simulink model "example"  (R2021a)
settings: Solver=VariableStepAuto  StartTime=0.0  StopTime=10.0  RelTol=1e-3
settings Model: Creator=ibirl  LastModifiedBy=zht

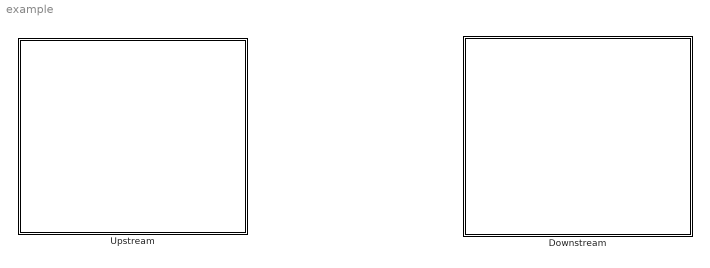
== system example ==
  Downstream : Stateflow chart  TreatAsAtomicUnit=on
  Upstream : Stateflow chart  TreatAsAtomicUnit=on

== stateflow chart example/Downstream ==
  state AFailed
  state BOperational
  state CStarved
  state DDelayed
  AFailed -> AFailed [order 3] : (1)[1-p3]{0}
  DDelayed -> AFailed [order 2] : (1)[p4]{0}
  AFailed -> CStarved [order 1] : (1)[p3*r2]{-1}
  AFailed -> BOperational [order 2] : (1)[p3*(1-r2)]{-1}
  BOperational -> AFailed [order 2] : (0)[p4*(1-r2)]{0}
  BOperational -> BOperational [order 3] : (1)[(1-p4)*(1-r2)]{-1}
  DDelayed -> BOperational [order 3] : (1)[(1-p4)*(1-q4)]{-1}
  BOperational -> CStarved [order 1] : (0)[r2]{-1}
  CStarved -> CStarved [order 2] : (1)[1-q3]{0}
  CStarved -> DDelayed [order 1] : (BOperational1)[q3]{0}
  DDelayed -> CStarved [order 1] : (1)[(1-p4)*q4]{-1}

== stateflow chart example/Upstream ==
  state AFailed
  state BOperational
  state CBlocked
  state DDelay
  AFailed -> AFailed [order 3] : (1)[1-p1]{0}
  DDelay -> AFailed [order 2] : (1)[p2]{0}
  AFailed -> CBlocked [order 1] : (1)[p1*r1]{1}
  AFailed -> BOperational [order 2] : (1)[p1*(1-r1)]{1}
  BOperational -> AFailed [order 2] : (0)[p2*(1-r1)]{0}
  BOperational -> BOperational [order 3] : (1)[(1-p2)*(1-r1)]{1}
  DDelay -> BOperational [order 3] : (1)[(1-p2)*(1-q2)]{1}
  BOperational -> CBlocked [order 1] : (0)[r1]{1}
  CBlocked -> CBlocked [order 2] : (1)[1-q1]{0}
  CBlocked -> DDelay [order 1] : (BOperational1)[q1]{0}
  DDelay -> CBlocked [order 1] : (1)[(1-p2)*q2]{1}
